simulink model "simulation"  (R2014b)
settings: Solver=ode45  StartTime=0.0  StopTime=400  RelTol=1e-3
libraries: simulink x1
settings Model: Creator=jonas  LastModifiedBy=jonas
settings DataIOCC: LimitDataPoints=off

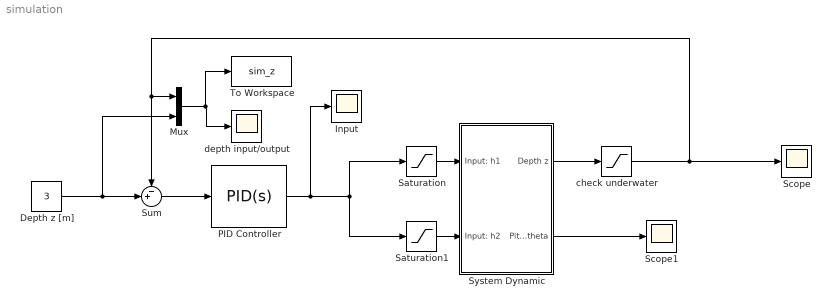
== system simulation ==
  Depth z [m] : Constant  Value=3
  Input : Scope
      settings: SaveName=ScopeData2
  Mux : Mux  Inputs=2
  PID Controller : simulink/Continuous/PID Controller  Controller=PID  TimeDomain=Continuous-time  SampleTime=-1  IntegratorMethod=Forward Euler  FilterMethod=Forward Euler  Form=Parallel  P=0.486312683438018  I=0.00382361167628227  D=5.61543108488242  N=2.12291335792304  InitialConditionSource=internal  InitialConditionForIntegrator=0  InitialConditionForFilter=0  ExternalReset=none  LimitOutput=on  UpperSaturationLimit=1  LowerSaturationLimit=0  LinearizeAsGain=on  AntiWindupMode=none  Kb=1  TrackingMode=off  Kt=1  PParamMin=[]  PParamMax=[]  IParamMin=[]  IParamMax=[]  DParamMin=[]  DParamMax=[]  NParamMin=[]  NParamMax=[]  KbParamMin=[]  KbParamMax=[]  KtParamMin=[]  KtParamMax=[]  POutMin=[]  POutMax=[]  IOutMin=[]  IOutMax=[]  DOutMin=[]  DOutMax=[]  NOutMin=[]  NOutMax=[]  KbOutMin=[]  KbOutMax=[]  KtOutMin=[]  KtOutMax=[]  IntegratorOutMin=[]  IntegratorOutMax=[]  FilterOutMin=[]  FilterOutMax=[]  SumOutMin=[]  SumOutMax=[]  SumI1OutMin=[]  SumI1OutMax=[]  SumI2OutMin=[]  SumI2OutMax=[]  SumI3OutMin=[]  SumI3OutMax=[]  SumDOutMin=[]  SumDOutMax=[]  SaturationOutMin=[]  SaturationOutMax=[]  IntegratorContinuousStateAttributes=''  IntegratorStateMustResolveToSignalObject=off  IntegratorRTWStateStorageClass=Auto  FilterContinuousStateAttributes=''  FilterStateMustResolveToSignalObject=off  FilterRTWStateStorageClass=Auto  DifferentiatorICPrevScaledInput=0  DifferentiatorOutMin=[]  DifferentiatorOutMax=[]  UseFilter=on
  Saturation : Saturate  UpperLimit=1  LowerLimit=0
  Saturation1 : Saturate  UpperLimit=1  LowerLimit=0
  Scope : Scope
  Scope1 : Scope
  Sum : Sum  Inputs=-+|
  System Dynamic : Subsystem
  To Workspace : ToWorkspace  VariableName=sim_z  SampleTime=0.01
  check underwater : Saturate  UpperLimit=1000  LowerLimit=0
  depth input/output : Scope
      settings: SaveName=ScopeData3
  wires:
  System Dynamic/1(Depth z) -> check underwater/1
  System Dynamic/2(Pitch theta) -> Scope1/1
  PID Controller/1 -> Input/1, Saturation1/1, Saturation/1
  Sum/1 -> PID Controller/1
  Mux/1 -> To Workspace/1, depth input/output/1
  Saturation/1 -> System Dynamic/1(Input: h1)
  Saturation1/1 -> System Dynamic/2(Input: h2)
  Depth z [m]/1 -> Mux/2, Sum/2
  check underwater/1 -> Mux/1, Sum/1, Scope/1

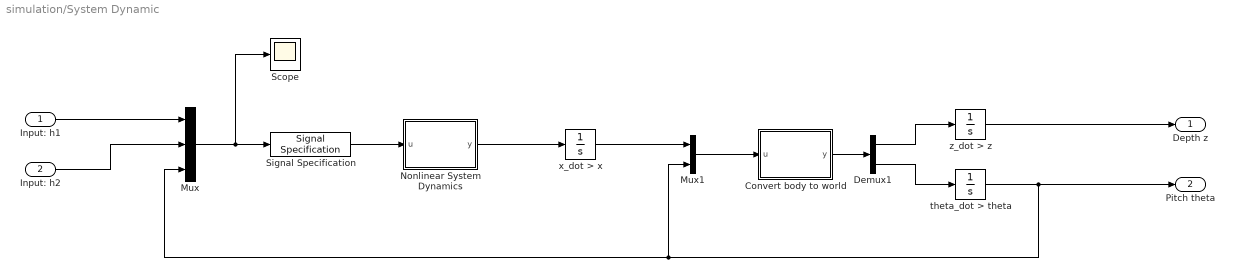
== system simulation/System Dynamic ==
  Input: h1 : Inport
  Input: h2 : Inport  Port=2
  Convert body to world : MATLAB Function  TreatAsAtomicUnit=on
  Demux1 : Demux  Outputs=2
  Mux : Mux  Inputs=3
  Mux1 : Mux  Inputs=2
  Nonlinear System Dynamics : MATLAB Function  TreatAsAtomicUnit=on
  Scope : Scope
      settings: SaveName=ScopeData4
  Signal Specification : SignalSpecification  Dimensions=3
  theta_dot > theta : Integrator
  x_dot > x : Integrator
  z_dot > z : Integrator
  Depth z : Outport
  Pitch theta : Outport  Port=2
  wires:
  Convert body to world/1(y) -> Demux1/1
  Demux1/1 -> z_dot > z/1
  Demux1/2 -> theta_dot > theta/1
  z_dot > z/1 -> Depth z/1
  theta_dot > theta/1 -> Mux1/2, Mux/3, Pitch theta/1
  Mux/1 -> Scope/1, Signal Specification/1
  Signal Specification/1 -> Nonlinear System Dynamics/1(u)
  Mux1/1 -> Convert body to world/1(u)
  x_dot > x/1 -> Mux1/1
  Nonlinear System Dynamics/1(y) -> x_dot > x/1
  Input: h1/1 -> Mux/1
  Input: h2/1 -> Mux/2

== matlab function simulation/System Dynamic/Convert body to world ==
  data: u input; y output
function y = fcn(u)

x_body = [u(1), u(2), u(3)]'; % [u, v, w]
theta = u(4);
% transform from body to earth frame
J = [-sin(theta), cos(theta), 0;...
    0, 0, 1];

y = J*x_body; % [z_dot, theta_dot]

== matlab function simulation/System Dynamic/Nonlinear System Dynamics ==
  data: u input; y output
function y = fcn(u)
%#codegen

% ---- PARAMETERS ----

g   = 9.81;                 % [m/s^2]   gravity
rho = 1000;                 % [kg/m^3]  density water

% parameters nanins specific
m0  = 12.5;                    % [kg]      empty weight Nanin
l_n = 0.4;                  % [m]       length Nanin
r_n = 0.1;                  % [m]       radius Nanin
V_n = r_n^2*pi*l_n;         % [m^3]     volume Nanin

x0_t = 0.25;                % [m]       displacement piston tank in x direction
z0_t = 0.05;                % [m]       displacement piston tank in z direction
A_t = pi*(65/(2*1000))^2;   % [m^2]     area piston tank
V_t = 250e-6;               % [m^3]     volume of piston tank
h_max = V_t/A_t;            % [m]       max height of water in piston tank

% restoring static forces
W_r = m0*g;          % [N]       gravitational force empty
B_r = rho*g*V_n;    % [N]       buoancy restoring force

% Added mass coefficents
Z_w = -rho*V_n;             % [kg]
M_q = -1/12*rho*V_n*l_n;    % [km*m]

% ------

% rename parameters for clarification
h1 = u(1);
h2 = u(2);
theta = u(3);

% Denormalize input
h1 = h1*h_max;
h2 = h2*h_max;

u_sys = [h1, h2]';

% calculate dynamic parameters
m = m0 + rho*A_t*(h1+h2); % dynamic mass
x1 = x0_t - h1/2;         % CoG of piston tank
x2 = -(x0_t - h2/2);
X_u = -0.1*m;

z_g = 0.005;
x_g = 0;
I_y = 0;

% calculate system model matrices
M = [m-X_u, 0,      m*z_g;...
     0,     m-Z_w,  -m*x_g;...
     m*z_g, -m*x_g, I_y-M_q];
 
g_static = [(W_r-B_r)*sin(theta);...
            -(W_r-B_r)*cos(theta);...
            z_g*W_r*sin(theta) + x_g*W_r*cos(theta)];
        
G_dyn = g*rho*A_t*[sin(theta),  sin(theta);...
                    -cos(theta), -cos(theta);...
                    sin(theta)*z0_t+cos(theta)*x1, sin(theta)*z0_t+cos(theta)*x2];
                
% calcuate state u_dot, w_dot, q_dot
x_dot = M\(-g_static -G_dyn*u_sys);

% return values
y = x_dot;
